simulink model "Sub_Vel_Pos_20180703"  (R2018a)
settings: Solver=VariableStepAuto  StartTime=0.0  StopTime=inf  RelTol=1e-3
libraries: robotlib x2
settings Model: Creator=F.Takuya  LastModifiedBy=Nishida-Lab

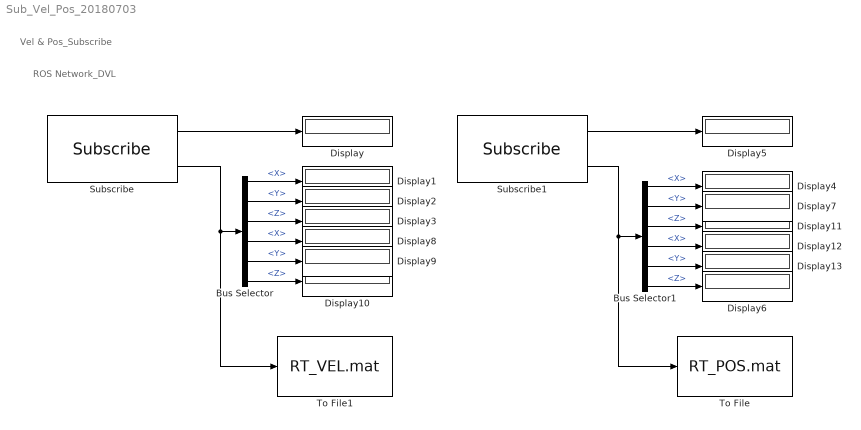
== system Sub_Vel_Pos_20180703 ==
  note: ROS Network_DVL
  note: Vel & Pos_Subscribe
  Bus Selector : BusSelector  OutputSignals=Twist.Linear.X,Twist.Linear.Y,Twist.Linear.Z,Twist.Angular.X,Twist.Angular.Y,Twist.Angular.Z
  Bus Selector1 : BusSelector  OutputSignals=Twist.Linear.X,Twist.Linear.Y,Twist.Linear.Z,Twist.Angular.X,Twist.Angular.Y,Twist.Angular.Z
  Display{,1..13} (14 alike) : Display
  Subscribe : robotlib/Subscribe  SourceLibraryInfo=This block requires Robotics System Toolbox  topicSource=Specify your own  topic=/RT_VEL  messageType=geometry_msgs/TwistStamped  sampleTime=-1  messageQueueLength=1
      settings: SourceProductBaseCode=RO
  Subscribe1 : robotlib/Subscribe  SourceLibraryInfo=This block requires Robotics System Toolbox  topicSource=Specify your own  topic=/RT_POS  messageType=geometry_msgs/TwistStamped  sampleTime=-1  messageQueueLength=1
      settings: SourceProductBaseCode=RO
  To File : ToFile  Filename=RT_POS.mat  MatrixName=RT_position  SaveFormat=Timeseries
  To File1 : ToFile  Filename=RT_VEL.mat  MatrixName=RT_velocity  SaveFormat=Timeseries
  wires:
  Subscribe/1 -> Display/1
  Subscribe1/1 -> Display5/1
  Subscribe/2 -> To File1/1, Bus Selector/1
  Bus Selector/1 -> Display1/1  "<X>"
  Bus Selector/2 -> Display2/1  "<Y>"
  Bus Selector/3 -> Display3/1  "<Z>"
  Bus Selector/4 -> Display8/1  "<X>"
  Bus Selector/5 -> Display9/1  "<Y>"
  Bus Selector/6 -> Display10/1  "<Z>"
  Bus Selector1/6 -> Display6/1  "<Z>"
  Subscribe1/2 -> Bus Selector1/1, To File/1
  Bus Selector1/2 -> Display7/1  "<Y>"
  Bus Selector1/5 -> Display13/1  "<Y>"
  Bus Selector1/4 -> Display12/1  "<X>"
  Bus Selector1/3 -> Display11/1  "<Z>"
  Bus Selector1/1 -> Display4/1  "<X>"
